simulink model "AUV_TopLevel"  (R2022b)
settings: Solver=ode4  StartTime=0.0  StopTime=300  FixedStep=0.01  RelTol=1e-3
undefined symbols (not defined in the file or in its folder): auv
settings Model: Creator=Abdullah Abdelaziz  LastModifiedBy=Abdullah Abdelaziz
settings DebuggingCC: AlgebraicLoopMsg=error

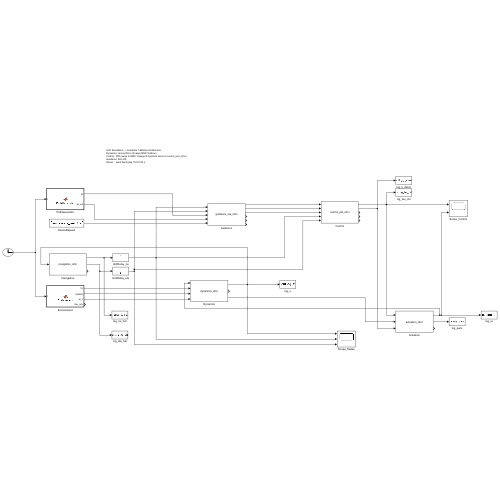
[thumbnail: Simulink's stored preview of the top-level diagram]
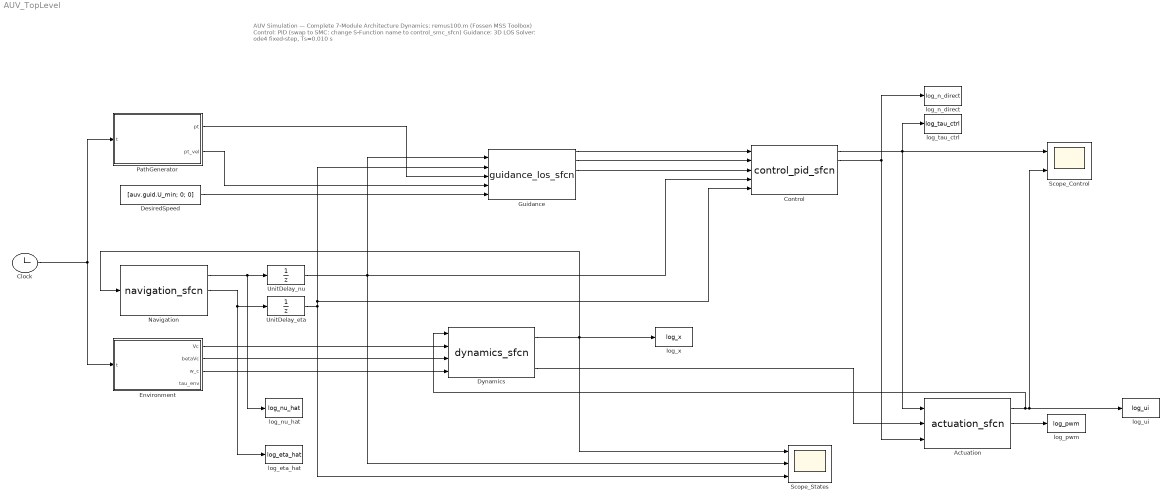
== system AUV_TopLevel ==
  note: AUV Simulation — Complete 7-Module Architecture
      | Dynamics: remus100.m (Fossen MSS Toolbox)
      | Control:  PID (swap to SMC: change S-Function name to control_smc_sfcn)
      | Guidance: 3D LOS
      | Solver:   ode4 fixed-step, Ts=0.010 s
  Actuation : M-S-Function  FunctionName=actuation_sfcn
  Clock : Clock
  Control : M-S-Function  FunctionName=control_pid_sfcn
  DesiredSpeed : Constant  Value=[auv.guid.U_min; 0; 0]
  Dynamics : M-S-Function  FunctionName=dynamics_sfcn
  Environment : MATLAB Function  TreatAsAtomicUnit=on
  Guidance : M-S-Function  FunctionName=guidance_los_sfcn
  Navigation : M-S-Function  FunctionName=navigation_sfcn
  PathGenerator : MATLAB Function  TreatAsAtomicUnit=on
  Scope_Control : Scope  NumInputPorts=2
  Scope_States : Scope  NumInputPorts=3
  UnitDelay_eta : UnitDelay  InitialCondition=zeros(6,1)  SampleTime=-1  HasFrameUpgradeWarning=on
  UnitDelay_nu : UnitDelay  InitialCondition=zeros(6,1)  SampleTime=-1  HasFrameUpgradeWarning=on
  log_eta_hat : ToWorkspace  VariableName=log_eta_hat  SampleTime=-1
  log_n_direct : ToWorkspace  VariableName=log_n_direct  SampleTime=-1
  log_nu_hat : ToWorkspace  VariableName=log_nu_hat  SampleTime=-1
  log_pwm : ToWorkspace  VariableName=log_pwm  SampleTime=-1
  log_tau_ctrl : ToWorkspace  VariableName=log_tau_ctrl  SampleTime=-1
  log_ui : ToWorkspace  VariableName=log_ui  SampleTime=-1
  log_x : ToWorkspace  VariableName=log_x  SampleTime=-1
  wires:
  DesiredSpeed/1 -> Guidance/5
  Clock/1 -> PathGenerator/1(t), Environment/1(t)
  PathGenerator/1(pt) -> Guidance/3
  PathGenerator/2(pt_vel) -> Guidance/4
  Environment/1(Vc) -> Dynamics/2
  Navigation/1 -> log_nu_hat/1, UnitDelay_nu/1
  Environment/2(betaVc) -> Dynamics/3
  Environment/3(w_c) -> Dynamics/4
  Guidance/1 -> Control/1
  Guidance/3 -> Control/3
  Guidance/2 -> Control/2
  Dynamics/1 -> log_x/1, Navigation/1, Scope_States/1
  Dynamics/3 -> Actuation/2
  Control/1 -> Scope_Control/1, log_tau_ctrl/1, Actuation/1
  Control/2 -> Actuation/3, log_n_direct/1
  Actuation/2 -> log_pwm/1
  Actuation/1 -> log_ui/1, Scope_Control/2, Dynamics/1
  UnitDelay_nu/1 -> Guidance/1, Control/4, Scope_States/2
  UnitDelay_eta/1 -> Guidance/2, Control/5, Scope_States/3
  Navigation/2 -> log_eta_hat/1, UnitDelay_eta/1

== matlab function AUV_TopLevel/PathGenerator ==
  data: t input; pt output; pt_vel output
function [pt, pt_vel] = PathGenerator(t)
% Queries the helix path at time t.
persistent path_data
if isempty(path_data)
    auv = evalin('base','auv');
    m=0.6; dt=auv.sim.Ts; T=auv.sim.T_end;
    time=0:dt:T; Yr=m*time;
    X=60*cos(0.02618*Yr); Y=60*sin(0.02618*Yr); Z=2+(2*Yr/200);
    dX=-60*0.02618*m*sin(0.02618*Yr);
    dY= 60*0.02618*m*cos(0.02618*Yr);
    dZ= 2*m/200*ones(size(time));
    path_data.pts=[X;Y;Z]; path_data.vel=[dX;dY;dZ];
    path_data.t_vec=time; path_data.T=T; path_data.dt=dt;
end
t_c = max(0, min(t, path_data.T));
idx = max(1, min(round(t_c/path_data.dt)+1, size(path_data.pts,2)));
pt     = path_data.pts(:,idx);
pt_vel = path_data.vel(:,idx);

== matlab function AUV_TopLevel/Environment ==
  data: t input; Vc output; betaVc output; w_c output; tau_env output
function [Vc, betaVc, w_c, tau_env] = Environment(t)
% Reads environment parameters from auv struct in base workspace.
auv = evalin('base','auv');
Vc     = auv.env.Vc_mean;
betaVc = auv.env.betaVc_mean;
w_c    = auv.env.w_c;
tau_env = zeros(6,1);
